simulink model "fxpdemo_feedback"  (Simulink 7.6)
settings: Solver=ode4  SolverMode=SingleTasking  StartTime=0.0  StopTime=4-2*0.01  FixedStep=0.01  RelTol=1e-3  AbsTol=1e-6
PostLoadFcn:
  | fxptdlg(bdroot(gcs))
Description:
  | Fixed-Point Tool
  | 
  | Upon opening, this model launches the Fixed-Point Tool.  The tool is a graphical user interface (GUI) that
  | automates common tasks of collecting min-max range data during simulations for use in automatically
  | selecting fixed-point scaling for blocks.  You can configure any fixed-point capable block in Simulink(R) to accept
  | the scaling proposed by the tool.  You can manually specify scaling for key blocks such as input ports and
  | selectively disable automated scaling in a model on a block-by-block basis.  This gives the Fixed-Point Tool more
  | information to work with and results in automatically selected fixed-point scalings that are compatible with the
  | key manually selected scalings.
settings Model: MinMaxOverflowLogging=MinMaxAndOverflow  Creator=The MathWorks Inc.  CovMetricSettings=d  ExtModeTrigMode=oneshot  ExtModeArmWhenConnect=off  ExtModeAutoUpdateStatusClock=off
settings SolverCC: InsertRTBMode=Auto
settings DataIOCC: LimitDataPoints=off  SaveFormat=StructureWithTime  SaveOutput=off  SaveTime=off  SignalLoggingName=sigsOut
settings OptimizationCC: InlineParams=on  InlineInvariantSignals=on  InitFltsAndDblsToZero=on
settings DebuggingCC: SaveWithParameterizedLinksMsg=none  SignalResolutionControl=TryResolveAllWithWarning  SolverPrmCheckMsg=none  MultiTaskDSMMsg=warning  MultiTaskCondExecSysMsg=none  SigSpecEnsureSampleTimeMsg=none  IntegerOverflowMsg=none  ParameterDowncastMsg=warning  ParameterOverflowMsg=warning  ParameterPrecisionLossMsg=none  StrictBusMsg=None  LoggingUnavailableSignals=none
settings HardwareCC: ProdHWDeviceType=Specified
settings RTWCC: GenerateReport=on  LaunchReport=on  IncludeERTFirstTime=on
settings CodeAppCC: GenerateComments=off  IncDataTypeInIds=on  SimulinkBlockComments=off
settings GRTTargetCC: TargetFcnLib=ansi_tfl_tmw.mat

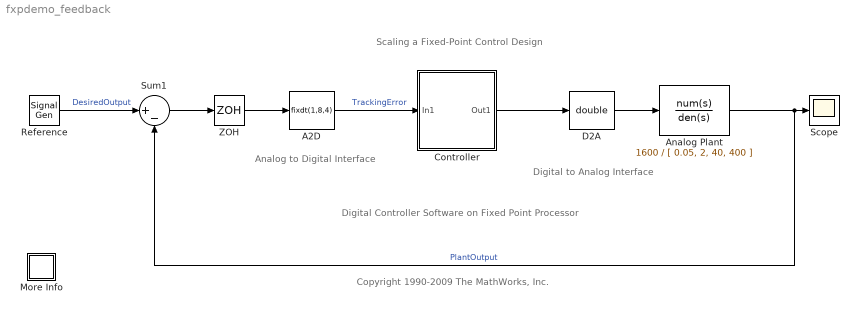
== system fxpdemo_feedback ==
  note: Analog to Digital
      | Interface
  note: Digital Controller
      | Software on
      | Fixed Point
      | Processor
  note: Digital to Analog
      | Interface
  note: Scaling a Fixed-Point Control Design
  note: Copyright 1990-2009 The MathWorks, Inc.
  A2D : DataTypeConversion  OutDataTypeStr=fixdt(1,8,4)  RndMeth=Nearest  SaturateOnIntegerOverflow=on  LockScale=on
  Analog Plant : TransferFcn  Numerator=1600  Denominator=[ 0.05, 2, 40, 400 ]
  Controller : Subsystem
  D2A : DataTypeConversion  OutDataTypeStr=double
  More Info : Subsystem
      settings: OpenFcn=showdemo(bdroot(gcs))
      mask Display: disp('?')
  Reference : SignalGenerator  WaveForm=square  Amplitude=2  Frequency=0.25
  Scope : Scope
      settings: TickLabels=on  YMin=-4  YMax=2.5  SaveName=PlantOutput
  Sum1 : Sum  Inputs=|+-  SaturateOnIntegerOverflow=on  InputSameDT=on  OutDataTypeStr=Inherit: Same as first input
  ZOH : ZeroOrderHold  SampleTime=0.01
  wires:
  A2D/1 -> Controller/1(In1)  "TrackingError"
  Controller/1(Out1) -> D2A/1
  ZOH/1 -> A2D/1
  Reference/1 -> Sum1/1  "DesiredOutput"
  D2A/1 -> Analog Plant/1
  Analog Plant/1 -> Scope/1, Sum1/2  "PlantOutput"
  Sum1/1 -> ZOH/1

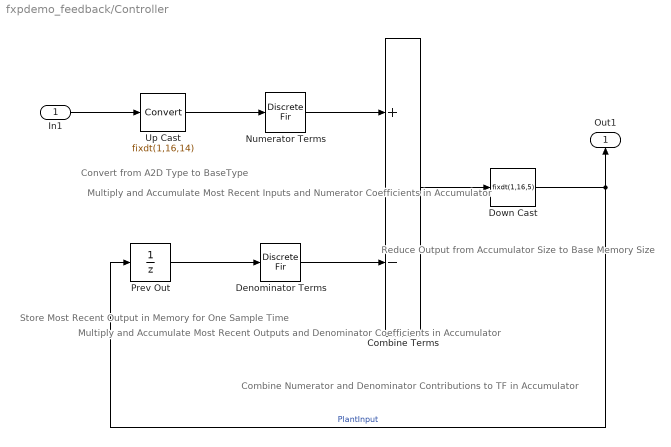
== system fxpdemo_feedback/Controller ==
  note: Convert from
      | A2D Type
      | to BaseType
  note: Multiply and Accumulate
      | Most Recent Inputs and
      | Numerator Coefficients
      | in Accumulator
  note: Multiply and Accumulate
      | Most Recent Outputs and
      | Denominator Coefficients
      | in Accumulator
  note: Store Most
      | Recent Output
      | in Memory for
      | One Sample Time
  note: Combine Numerator
      | and Denominator
      | Contributions to TF
      | in Accumulator
  note: Reduce Output from
      | Accumulator Size to
      | Base Memory Size
  In1 : Inport
  Combine Terms : Sum  Inputs=+-  OutDataTypeStr=fixdt(1,32,12)  SaturateOnIntegerOverflow=on
  Denominator Terms : DiscreteFir  NumCoeffs=[ -1.968253968253968, 1.247165532879818, -0.2993197278911561, 0.02040816326530606 ]  IC=0.0  SampleTime=0.01  CoefDataTypeStr=fixdt(1,16)  ProductDataTypeStr=fixdt(1,32,12)  AccumDataTypeStr=fixdt(1,32,12)  OutDataTypeStr=fixdt(1,32,12)  SaturateOnIntegerOverflow=on
  Down Cast : DataTypeConversion  OutDataTypeStr=fixdt(1,16,5)  SaturateOnIntegerOverflow=on
  Numerator Terms : DiscreteFir  NumCoeffs=[ 0.8859903814981437, -1.419326114832407, -0.2858969781410884, 1.425131129616998, -0.5942883885724647 ]  IC=0.0  SampleTime=0.01  CoefDataTypeStr=fixdt(1,16)  ProductDataTypeStr=fixdt(1,32,12)  AccumDataTypeStr=fixdt(1,32,12)  OutDataTypeStr=fixdt(1,32,12)  SaturateOnIntegerOverflow=on
  Prev Out : UnitDelay  X0=0.0  SampleTime=0.01
  Up Cast : DataTypeConversion  OutDataTypeStr=fixdt(1,16,14)  SaturateOnIntegerOverflow=on
  Out1 : Outport  InitialOutput=0
  wires:
  Combine Terms/1 -> Down Cast/1
  Denominator Terms/1 -> Combine Terms/2
  Numerator Terms/1 -> Combine Terms/1
  Prev Out/1 -> Denominator Terms/1
  Up Cast/1 -> Numerator Terms/1
  In1/1 -> Up Cast/1
  Down Cast/1 -> Prev Out/1, Out1/1  "PlantInput"

== system fxpdemo_feedback/More Info ==
